simulink model "Q1_Lotka_Volterra"  (R2026a)
settings: Solver=ode45  StopTime=25  RelTol=1e-8  AbsTol=1e-10
settings Model: Creator=szj  LastModifiedBy=szj

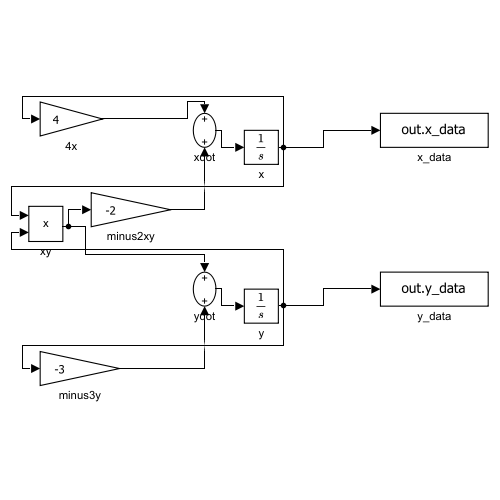
[thumbnail: Simulink's stored preview of the top-level diagram]
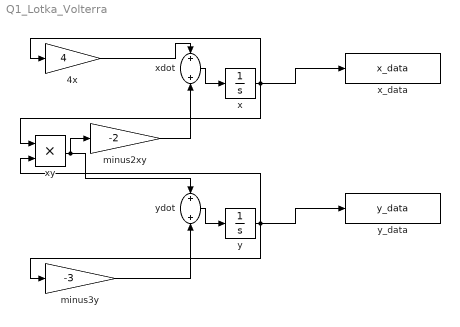
== system Q1_Lotka_Volterra ==
  4x : Gain  Gain=4
  minus2xy : Gain  Gain=-2
  minus3y : Gain  Gain=-3
  x : Integrator  InitialCondition=2
  x_data : ToWorkspace  VariableName=x_data  SaveFormat=Timeseries  SampleTime=-1
  xdot : Sum
  xy : Product
  y : Integrator  InitialCondition=3
  y_data : ToWorkspace  VariableName=y_data  SaveFormat=Timeseries  SampleTime=-1
  ydot : Sum
  wires:
  x/1 -> 4x/1, xy/1, x_data/1
  y/1 -> xy/2, minus3y/1, y_data/1
  xy/1 -> minus2xy/1, ydot/1
  4x/1 -> xdot/1
  minus2xy/1 -> xdot/2
  minus3y/1 -> ydot/2
  xdot/1 -> x/1
  ydot/1 -> y/1
